simulink model "tuto2"  (R2016a)
settings: Solver=VariableStepAuto  StartTime=0.0  StopTime=20  RelTol=1e-3
undefined symbols (not defined in the file): PosInit, VitesseInit
libraries: simulink x1
settings Model: Creator=nsurbayr  LastModifiedBy=nsurbayr

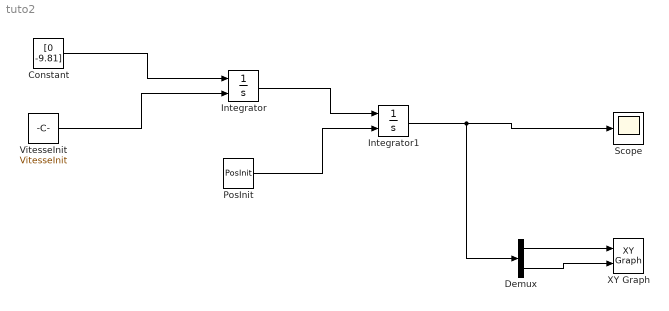
== system tuto2 ==
  Constant : Constant  Value=[0 -9.81]
  Demux : Demux  Outputs=2
  Integrator : Integrator  InitialConditionSource=external
  Integrator1 : Integrator  InitialConditionSource=external
  PosInit : Constant  Value=PosInit
  Scope : Scope
  "VitesseInit " : Constant  Value=VitesseInit
  XY Graph : simulink/Sinks/XY Graph  xmin=-1  xmax=20  ymin=-500  ymax=200  st=-1
  wires:
  Constant/1 -> Integrator/1
  Integrator/1 -> Integrator1/1
  "VitesseInit "/1 -> Integrator/2
  PosInit/1 -> Integrator1/2
  Integrator1/1 -> Demux/1, Scope/1
  Demux/2 -> XY Graph/2
  Demux/1 -> XY Graph/1
